simulink model "closed_loop_estimation"  (R2023a)
settings: Solver=FixedStepAuto  StartTime=start_time  StopTime=stop_time  FixedStep=sample_time  RelTol=1e-3
values from neighbouring files (symbols this model uses):
  a = -0.8    [example12.m]    (also in example14.m; example15.m; example16.m)
  b = 0.5    [example12.m]    (also in example14.m; example15.m; example16.m)
  c = -0.5    [example12.m]    (also in example14.m = 0; example15.m = 0; example16.m = 0)
  K = [0.2, 0.32]    [example14.m]
  mean_e = 0    [example12.m]    (also in example14.m; example15.m)
  P0 = 100 * eye(3)    [example12.m]    (also in example14.m = 0.01 * eye(2); example15.m = 100 * eye(2); example16.m = 0.01)
  sample_time = 1    [example12.m]    (also in example14.m; example15.m; example16.m)
  seed_e = 6    [example12.m]    (also in example14.m = i; example15.m = 2)
  std_e = 0.5    [example12.m]    (also in example14.m; example15.m)
  theta0 = zeros(3,1)    [example12.m]    (also in example14.m = Theta(:,i); example15.m = zeros(2,1); example16.m = zeros(n_phi, 1))
  y0 = 0    [example14.m]    (also in example15.m)
Description:
  | Estimate model parameter with RLS when input generate throug the feedback.
settings Model: Creator=Beigi  LastModifiedBy=Mmoha

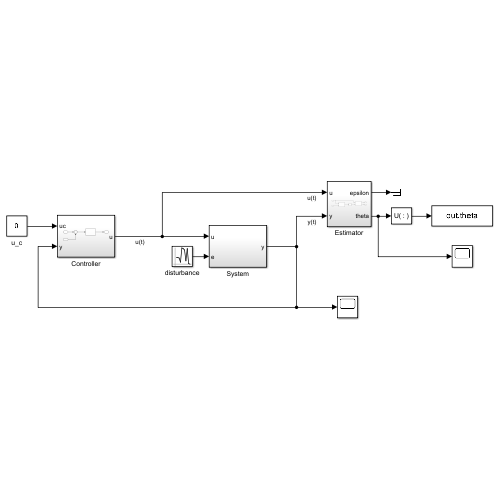
[thumbnail: Simulink's stored preview of the top-level diagram]
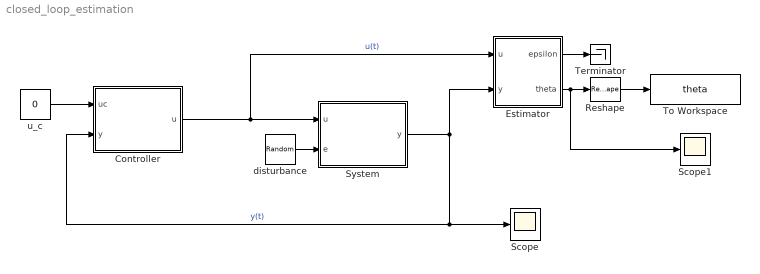
== system closed_loop_estimation ==
  Controller : Subsystem
  Estimator : Subsystem
  Reshape : Reshape
  Scope : Scope
  Scope1 : Scope
  System : Subsystem
  Terminator : Terminator
  To Workspace : ToWorkspace  VariableName=theta  SaveFormat=Timeseries  SampleTime=-1
  disturbance : RandomNumber  Mean=mean_e  Variance=std_e^2  Seed=seed_e  SampleTime=sample_time
  u_c : Constant  Value=0
  wires:
  disturbance/1 -> System/2(e)
  Controller/1(u) -> Estimator/1(u), System/1(u)  "u(t)"
  System/1(y) -> Estimator/2(y), Scope/1, Controller/2(y)  "y(t)"
  u_c/1 -> Controller/1(uc)
  Estimator/1(epsilon) -> Terminator/1
  Estimator/2(theta) -> Scope1/1, Reshape/1
  Reshape/1 -> To Workspace/1

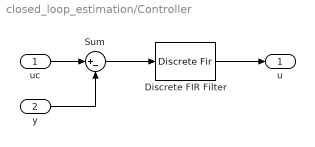
== system closed_loop_estimation/Controller ==
  uc : Inport
  y : Inport  Port=2
  Discrete FIR Filter : DiscreteFir  Coefficients=K
  Sum : Sum  Inputs=|+-
  u : Outport
  wires:
  uc/1 -> Sum/1
  y/1 -> Sum/2
  Discrete FIR Filter/1 -> u/1
  Sum/1 -> Discrete FIR Filter/1

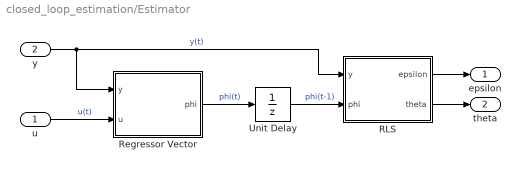
== system closed_loop_estimation/Estimator ==
  u : Inport
  y : Inport  Port=2
  RLS : Subsystem
  Regressor Vector : Subsystem
  Unit Delay : UnitDelay  SampleTime=-1  HasFrameUpgradeWarning=on
  epsilon : Outport
  theta : Outport  Port=2
  wires:
  u/1 -> Regressor Vector/2(u)  "u(t)"
  Regressor Vector/1(phi) -> Unit Delay/1  "phi(t)"
  y/1 -> Regressor Vector/1(y), RLS/1(y)  "y(t)"
  Unit Delay/1 -> RLS/2(phi)  "phi(t-1)"
  RLS/2(theta) -> theta/1
  RLS/1(epsilon) -> epsilon/1

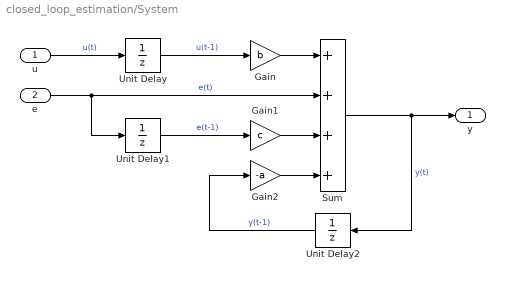
== system closed_loop_estimation/System ==
  u : Inport
  e : Inport  Port=2
  Gain : Gain  Gain=b
  Gain1 : Gain  Gain=c
  Gain2 : Gain  Gain=-a
  Sum : Sum  Inputs=++++
  Unit Delay : UnitDelay  SampleTime=-1  HasFrameUpgradeWarning=on
  Unit Delay1 : UnitDelay  SampleTime=-1  HasFrameUpgradeWarning=on
  Unit Delay2 : UnitDelay  InitialCondition=y0  SampleTime=-1  HasFrameUpgradeWarning=on
  y : Outport
  wires:
  u/1 -> Unit Delay/1  "u(t)"
  Unit Delay/1 -> Gain/1  "u(t-1)"
  Gain/1 -> Sum/1
  e/1 -> Unit Delay1/1, Sum/2  "e(t)"
  Unit Delay1/1 -> Gain1/1  "e(t-1)"
  Gain1/1 -> Sum/3
  Sum/1 -> Unit Delay2/1, y/1  "y(t)"
  Gain2/1 -> Sum/4
  Unit Delay2/1 -> Gain2/1  "y(t-1)"

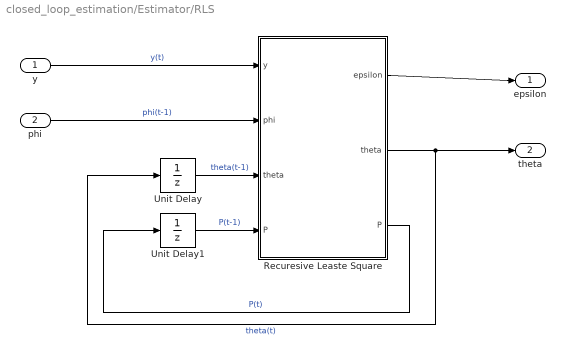
== system closed_loop_estimation/Estimator/RLS ==
  y : Inport
  phi : Inport  Port=2
  Recuresive Leaste Square : MATLAB Function  TreatAsAtomicUnit=on
  Unit Delay : UnitDelay  InitialCondition=theta0  SampleTime=-1  HasFrameUpgradeWarning=on
  Unit Delay1 : UnitDelay  InitialCondition=P0  SampleTime=-1  HasFrameUpgradeWarning=on
  epsilon : Outport
  theta : Outport  Port=2
  wires:
  y/1 -> Recuresive Leaste Square/1(y)  "y(t)"
  phi/1 -> Recuresive Leaste Square/2(phi)  "phi(t-1)"
  Unit Delay/1 -> Recuresive Leaste Square/3("theta ")  "theta(t-1)"
  Unit Delay1/1 -> Recuresive Leaste Square/4("P ")  "P(t-1)"
  Recuresive Leaste Square/3(P) -> Unit Delay1/1  "P(t)"
  Recuresive Leaste Square/2(theta) -> theta/1, Unit Delay/1  "theta(t)"
  Recuresive Leaste Square/1(epsilon) -> epsilon/1

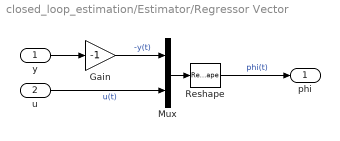
== system closed_loop_estimation/Estimator/Regressor Vector ==
  y : Inport
  u : Inport  Port=2
  Gain : Gain  Gain=-1
  Mux : Mux  Inputs=2
  Reshape : Reshape  OutputDimensionality=Column vector (2-D)
  phi : Outport
  wires:
  y/1 -> Gain/1
  Mux/1 -> Reshape/1
  Gain/1 -> Mux/1  "-y(t)"
  u/1 -> Mux/2  "u(t)"
  Reshape/1 -> phi/1  "phi(t)"

== matlab function closed_loop_estimation/Estimator/RLS/Recuresive Leaste Square ==
  data: y input size=1; epsilon output size=1; phi input size=[2, 1]; theta input size=[2, 1]; P input size=[2, 2]; theta output; P output
function [epsilon, theta, P] = RLS(y,phi,theta,P)
epsilon = y - phi' * theta;
P = P - P * phi / ( 1 + phi' * P * phi ) * phi' * P;
theta = theta + P * phi * epsilon;
